simulink model "export_archive_task"  (Simulink 3.00)
libraries: arclib x4, mathlib x2, genlib x2

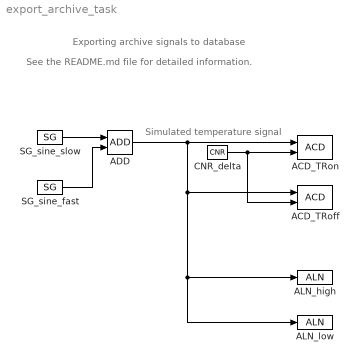
== system export_archive_task ==
  note: See the README.md file for detailed information.
  note: Exporting archive signals to database
  note: Simulated temperature signal
  ACD_TRoff : arclib/ACD  acls=8: Double  arc=1  id=2  tmin=0.1  tmax=5  TR=off  Desc=Simulated temperature signal, TR=off
  ACD_TRon : arclib/ACD  acls=8: Double  arc=1  id=1  tmin=0.1  tmax=5  TR=on  Desc=Simulated temperature signal, TR=on
  ADD : mathlib/ADD
  ALN_high : arclib/ALN  hys=0.5  hh=5e10  h=11  l=0  ll=-5e10  acls=8: Double  arc=1  id=52  lvl1=33  lvl2=43  Desc=Value too high!  iACK=4
  ALN_low : arclib/ALN  hys=0.5  hh=5e10  h=0  l=-7.5  ll=-5e10  acls=8: Double  arc=1  id=53  lvl1=32  lvl2=42  Desc=Value too low!  iACK=2
  CNR_delta : mathlib/CNR  ycn=0.2
  SG_sine_fast : genlib/SG  isig=1: SINE  amp=3  freq=0.09  phase=0  ifrunit=1: Hz  iphunit=1: degrees  offset=0
  SG_sine_slow : genlib/SG  isig=1: SINE  amp=10  freq=0.025  phase=0  ifrunit=1: Hz  iphunit=1: degrees  offset=0
  wires:
  ADD/1 -> ACD_TRon/1, ACD_TRoff/1, ALN_high/1, ALN_low/1
  CNR_delta/1 -> ACD_TRoff/2, ACD_TRon/2
  SG_sine_fast/1 -> ADD/2
  SG_sine_slow/1 -> ADD/1
